simulink model "SIM_response_pr_L_nu_gap"  (Simulink 7.9)
settings: Solver=ode4  StartTime=0.0  StopTime=2  FixedStep=10e-5  RelTol=1e-3
undefined symbols (not defined in the file or in its folder): CI
settings Model: Creator=jingxuan  LastModifiedBy=jingxuan

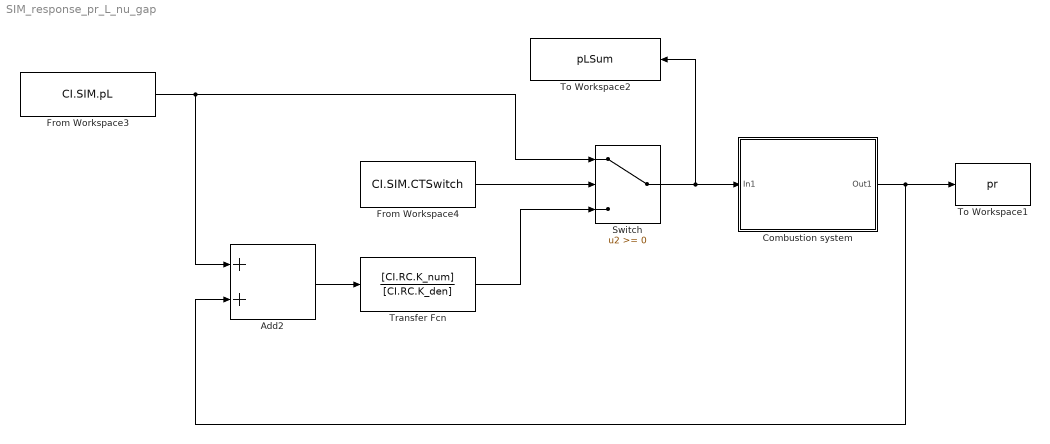
== system SIM_response_pr_L_nu_gap ==
  Add2 : Sum
  Combustion system : Subsystem
  From Workspace3 : FromWorkspace  VariableName=CI.SIM.pL  SampleTime=0
  From Workspace4 : FromWorkspace  VariableName=CI.SIM.CTSwitch  SampleTime=0
  Switch : Switch
  To Workspace1 : ToWorkspace  VariableName=pr  SampleTime=-1
  To Workspace2 : ToWorkspace  VariableName=pLSum  SampleTime=-1
  Transfer Fcn : TransferFcn  Numerator=[CI.RC.K_num]  Denominator=[CI.RC.K_den]
  wires:
  Combustion system/1(Out1) -> To Workspace1/1, Add2/2
  Switch/1 -> Combustion system/1(In1), To Workspace2/1
  From Workspace3/1 -> Switch/1, Add2/1
  From Workspace4/1 -> Switch/2
  Transfer Fcn/1 -> Switch/3
  Add2/1 -> Transfer Fcn/1

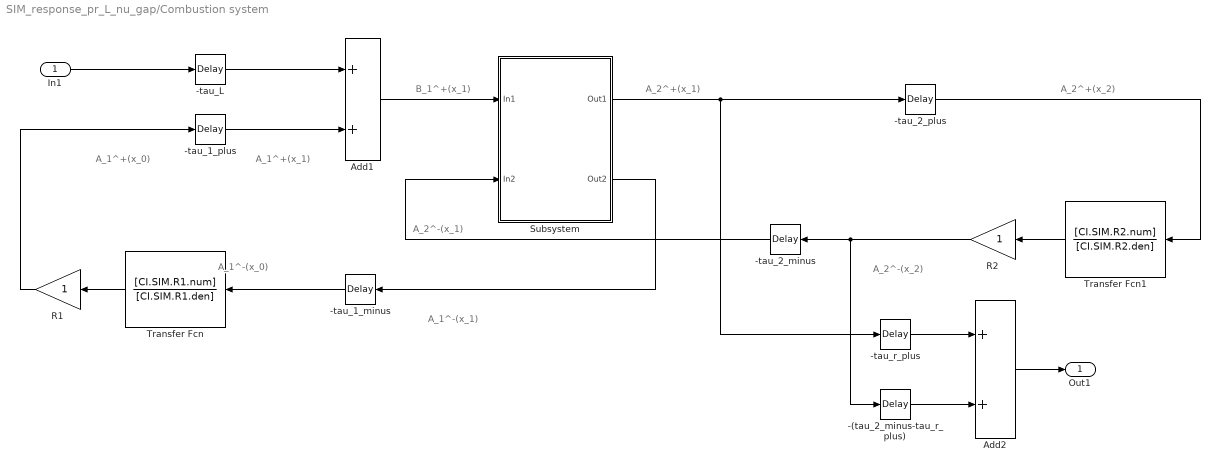
== system SIM_response_pr_L_nu_gap/Combustion system ==
  note: A_2^+(x_1)
  note: A_1^-(x_0)
  note: A_1^+(x_0)
  note: A_1^+(x_1)
  note: A_2^+(x_2)
  note: A_2^-(x_2)
  note: B_1^+(x_1)
  note: A_2^-(x_1)
  note: A_1^-(x_1)
  In1 : Inport
  -(tau_2_minus-tau_r_plus) : TransportDelay  DelayTime=CI.SIM.tauMMic  BufferSize=65536
  -tau_1_minus : TransportDelay  DelayTime=CI.TP.tau_minus(1) + CI.SIM.R1.tau  BufferSize=65536
  -tau_1_plus : TransportDelay  DelayTime=CI.TP.tau_plus(1)  BufferSize=65536
  -tau_2_minus : TransportDelay  DelayTime=CI.TP.tau_minus(2)  BufferSize=65536
  -tau_2_plus : TransportDelay  DelayTime=CI.TP.tau_plus(2) + CI.SIM.R2.tau  BufferSize=65536
  -tau_L : TransportDelay  DelayTime=CI.TP.tau_plus(1)  BufferSize=65536
  -tau_r_plus : TransportDelay  DelayTime=CI.SIM.tauPMic  BufferSize=65536
  Add1 : Sum
  Add2 : Sum
  R1 : Gain
  R2 : Gain
  Subsystem : Subsystem
  Transfer Fcn : TransferFcn  Numerator=[CI.SIM.R1.num]  Denominator=[CI.SIM.R1.den]
  Transfer Fcn1 : TransferFcn  Numerator=[CI.SIM.R2.num]  Denominator=[CI.SIM.R2.den]
  Out1 : Outport
  wires:
  -tau_L/1 -> Add1/1
  R1/1 -> -tau_1_plus/1
  -tau_1_plus/1 -> Add1/2
  -tau_2_minus/1 -> Subsystem/2(In2)
  -tau_r_plus/1 -> Add2/1
  R2/1 -> -tau_2_minus/1, -(tau_2_minus-tau_r_plus)/1
  Subsystem/1(Out1) -> -tau_2_plus/1, -tau_r_plus/1
  Add1/1 -> Subsystem/1(In1)
  Subsystem/2(Out2) -> -tau_1_minus/1
  -(tau_2_minus-tau_r_plus)/1 -> Add2/2
  In1/1 -> -tau_L/1
  Add2/1 -> Out1/1
  -tau_1_minus/1 -> Transfer Fcn/1
  Transfer Fcn1/1 -> R2/1
  -tau_2_plus/1 -> Transfer Fcn1/1
  Transfer Fcn/1 -> R1/1

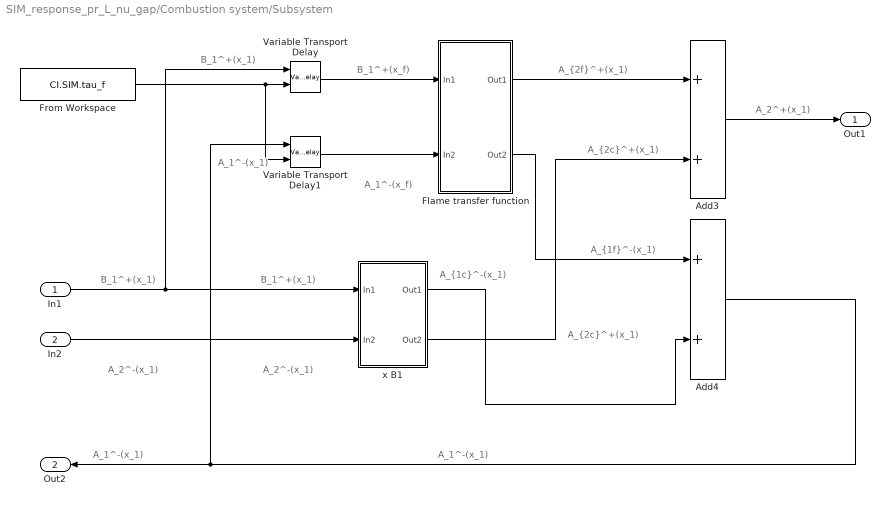
== system SIM_response_pr_L_nu_gap/Combustion system/Subsystem ==
  note: B_1^+(x_1)
  note: A_1^-(x_1)
  note: A_1^-(x_f)
  note: B_1^+(x_f)
  note: B_1^+(x_1)
  note: A_2^-(x_1)
  note: A_1^-(x_1)
  note: A_1^-(x_1)
  note: A_2^+(x_1)
  note: B_1^+(x_1)
  note: A_2^-(x_1)
  note: A_{2f}^+(x_1)
  note: A_{2c}^+(x_1)
  note: A_{2c}^+(x_1)
  note: A_{1c}^-(x_1)
  note: A_{1f}^-(x_1)
  In1 : Inport
  In2 : Inport  Port=2
  Add3 : Sum
  Add4 : Sum
  Flame transfer function : Subsystem
  From Workspace : FromWorkspace  VariableName=CI.SIM.tau_f  SampleTime=0
  Variable Transport Delay : VariableTransportDelay  VariableDelayType=Variable transport delay  MaximumDelay=0.01
  Variable Transport Delay1 : VariableTransportDelay  VariableDelayType=Variable transport delay  MaximumDelay=0.01
  x B1 : Subsystem
  Out1 : Outport
  Out2 : Outport  Port=2
  wires:
  In1/1 -> x B1/1(In1), Variable Transport Delay/1
  Flame transfer function/1(Out1) -> Add3/1
  Add4/1 -> Out2/1, Variable Transport Delay1/1
  Flame transfer function/2(Out2) -> Add4/1
  Add3/1 -> Out1/1
  In2/1 -> x B1/2(In2)
  Variable Transport Delay/1 -> Flame transfer function/1(In1)
  From Workspace/1 -> Variable Transport Delay/2, Variable Transport Delay1/2
  Variable Transport Delay1/1 -> Flame transfer function/2(In2)
  x B1/2(Out2) -> Add3/2
  x B1/1(Out1) -> Add4/2

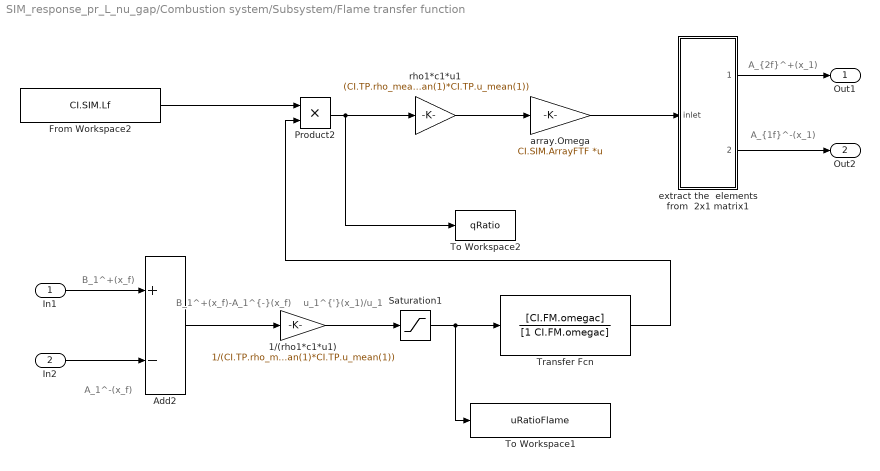
== system SIM_response_pr_L_nu_gap/Combustion system/Subsystem/Flame transfer function ==
  note: A_1^-(x_f)
  note: B_1^+(x_f)
  note: A_{2f}^+(x_1)
  note: A_{1f}^-(x_1)
  note: u_1^{'}(x_1)/u_1
  note: B_1^+(x_f)-A_1^{-}(x_f)
  In1 : Inport
  In2 : Inport  Port=2
  1/(rho1*c1*u1) : Gain  Gain=1/(CI.TP.rho_mean(1)*CI.TP.c_mean(1)*CI.TP.u_mean(1))
  Add2 : Sum  Inputs=+-
  From Workspace2 : FromWorkspace  VariableName=CI.SIM.Lf  SampleTime=0
  Product2 : Product  RndMeth=Zero
  Saturation1 : Saturate  UpperLimit=CI.SIM.epsilon_max  LowerLimit=-CI.SIM.epsilon_max
  To Workspace1 : ToWorkspace  VariableName=uRatioFlame  SampleTime=-1
  To Workspace2 : ToWorkspace  VariableName=qRatio  SampleTime=-1
  Transfer Fcn : TransferFcn  Numerator=[CI.FM.omegac]  Denominator=[1 CI.FM.omegac]
  array.Omega : Gain  Gain=CI.SIM.ArrayFTF  Multiplication=Matrix(K*u)
  extract the  elements from  2x1 matrix1 : Subsystem
  rho1*c1*u1 : Gain  Gain=(CI.TP.rho_mean(1)*CI.TP.c_mean(1)*CI.TP.u_mean(1))
  Out1 : Outport
  Out2 : Outport  Port=2
  wires:
  In1/1 -> Add2/1
  extract the  elements from  2x1 matrix1/1(outlet 1) -> Out1/1
  In2/1 -> Add2/2
  extract the  elements from  2x1 matrix1/2(outlet 2) -> Out2/1
  Add2/1 -> 1/(rho1*c1*u1)/1
  1/(rho1*c1*u1)/1 -> Saturation1/1
  Saturation1/1 -> To Workspace1/1, Transfer Fcn/1
  From Workspace2/1 -> Product2/1
  Product2/1 -> rho1*c1*u1/1, To Workspace2/1
  array.Omega/1 -> extract the  elements from  2x1 matrix1/1(inlet)
  rho1*c1*u1/1 -> array.Omega/1
  Transfer Fcn/1 -> Product2/2

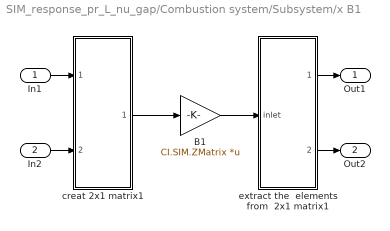
== system SIM_response_pr_L_nu_gap/Combustion system/Subsystem/x B1 ==
  In1 : Inport
  In2 : Inport  Port=2
  B1 : Gain  Gain=CI.SIM.ZMatrix  Multiplication=Matrix(K*u)
  creat 2x1 matrix1 : Subsystem
  extract the  elements from  2x1 matrix1 : Subsystem
  Out1 : Outport
  Out2 : Outport  Port=2
  wires:
  creat 2x1 matrix1/1("outlet ") -> B1/1
  B1/1 -> extract the  elements from  2x1 matrix1/1(inlet)
  In1/1 -> creat 2x1 matrix1/1(inlet 1)
  extract the  elements from  2x1 matrix1/1(outlet 1) -> Out1/1
  In2/1 -> creat 2x1 matrix1/2(inlet 2)
  extract the  elements from  2x1 matrix1/2(outlet 2) -> Out2/1

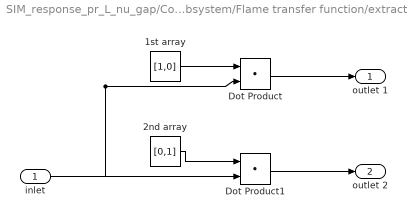
== system SIM_response_pr_L_nu_gap/Combustion system/Subsystem/Flame transfer function/extract the  elements from  2x1 matrix1 ==
  inlet : Inport
  1st array : Constant  Value=[1,0]  VectorParams1D=off
  2nd array : Constant  Value=[0,1]  VectorParams1D=off
  Dot Product : DotProduct  InputSameDT=on  OutDataTypeStr=Inherit: Inherit via internal rule
  Dot Product1 : DotProduct  InputSameDT=on  OutDataTypeStr=Inherit: Inherit via internal rule
  outlet 1 : Outport
  outlet 2 : Outport  Port=2
  wires:
  1st array/1 -> Dot Product/1
  2nd array/1 -> Dot Product1/1
  Dot Product/1 -> outlet 1/1
  Dot Product1/1 -> outlet 2/1
  inlet/1 -> Dot Product/2, Dot Product1/2

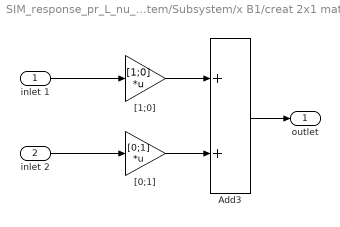
== system SIM_response_pr_L_nu_gap/Combustion system/Subsystem/x B1/creat 2x1 matrix1 ==
  inlet 1 : Inport
  inlet 2 : Inport  Port=2
  Add3 : Sum
  "[0;1]" : Gain  Gain=[0;1]  Multiplication=Matrix(K*u)
  "[1;0]" : Gain  Gain=[1;0]  Multiplication=Matrix(K*u)
  "outlet " : Outport
  wires:
  inlet 1/1 -> "[1;0]"/1
  inlet 2/1 -> "[0;1]"/1
  "[1;0]"/1 -> Add3/1
  "[0;1]"/1 -> Add3/2
  Add3/1 -> "outlet "/1

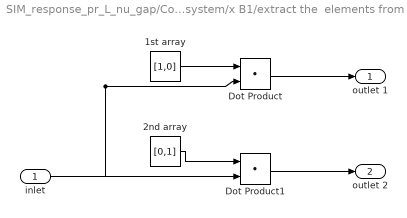
== system SIM_response_pr_L_nu_gap/Combustion system/Subsystem/x B1/extract the  elements from  2x1 matrix1 ==
  inlet : Inport
  1st array : Constant  Value=[1,0]  VectorParams1D=off
  2nd array : Constant  Value=[0,1]  VectorParams1D=off
  Dot Product : DotProduct  InputSameDT=on  OutDataTypeStr=Inherit: Inherit via internal rule
  Dot Product1 : DotProduct  InputSameDT=on  OutDataTypeStr=Inherit: Inherit via internal rule
  outlet 1 : Outport
  outlet 2 : Outport  Port=2
  wires:
  1st array/1 -> Dot Product/1
  2nd array/1 -> Dot Product1/1
  Dot Product/1 -> outlet 1/1
  Dot Product1/1 -> outlet 2/1
  inlet/1 -> Dot Product/2, Dot Product1/2
